simulink model "ABS_simp"  (R2015a)
settings: Solver=FixedStepDiscrete  StartTime=0.0  StopTime=1.0  FixedStep=1.0  RelTol=1e-3
libraries: simulink x2
settings Model: Creator=Teme  LastModifiedBy=Teme
settings DataIOCC: ExternalInput=Inputs_Safety_1_01062016175621  LoadExternalInput=on  SaveFormat=Structure  SaveState=on
settings RTWCC: Toolchain=Clang v3.1 | gmake (64-bit Mac)
settings GRTTargetCC: ExtMode=on

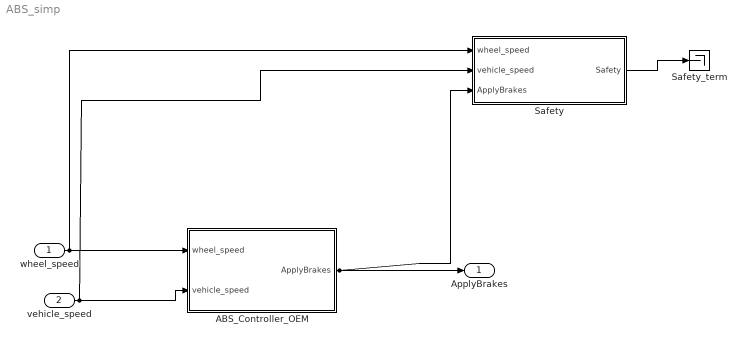
== system ABS_simp ==
  wheel_speed : Inport  SampleTime=0
  vehicle_speed : Inport  Port=2  SampleTime=0
  ABS_Controller_OEM : Subsystem
  Safety : Subsystem  TreatAsAtomicUnit=on  mask(Observer){AnnotationType=ensures, ObserverType=[]}
      mask prompts: AnnotationType "Type of annotation (pre/post...)"; ObserverType "Observer type"
      mask help:
      | Set an observer for the system.
      | The annotation type parameter sets the type of observer:
      | - requires : pre-condition
      | - ensures : post-condition
      | - assert : an assertion
      | - observer : the observer computes a special type of properties
      mask TypeOptions AnnotationType: ensures | requires | assert | observer
      mask Callback AnnotationType:
      | paramStr = get_param(gcb, 'MaskValues');
      | if strcmp(paramStr{1}(1),'o')
      | set_param(gcb,'MaskVisibilities',{'on';'on'});
      | paramStr{2} = 'ellipsoid';
      | set_param(gcb,'MaskValues',paramStr);
      | else
      | set_param(gcb,'MaskVisibilities',{'on';'off'});
      | end
      | clear paramStr;
      mask Callback ObserverType:
      | paramStr = get_param(gcb, 'MaskValues');
      | if strcmp(paramStr{1}(1),'o')
      | set_param(gcb,'MaskVisibilities',{'on';'on'});
      | paramStr{2} = 'ellipsoid';
      | set_param(gcb,'MaskValues',paramStr);
      | else
      | set_param(gcb,'MaskVisibilities',{'on';'off'});
      | end
      | clear paramStr;
      mask Display:
      | color('red')
      | text(0.5, 0.5, ['CoCoSpec: ''' get_param(gcb,'name') ''''], 'horizontalAlignment', 'center');
      | text(0.99, 0.03, '{\bf\fontsize{12}TO BE VERIFIED}', 'hor', 'right', 'ver', 'bottom', 'texmode', 'on');
  Safety_term : Terminator
  ApplyBrakes : Outport
  wires:
  wheel_speed/1 -> ABS_Controller_OEM/1(wheel_speed), Safety/1(wheel_speed)
  vehicle_speed/1 -> ABS_Controller_OEM/2(vehicle_speed), Safety/2(vehicle_speed)
  ABS_Controller_OEM/1(ApplyBrakes) -> ApplyBrakes/1, Safety/3(ApplyBrakes)
  Safety/1(Safety) -> Safety_term/1

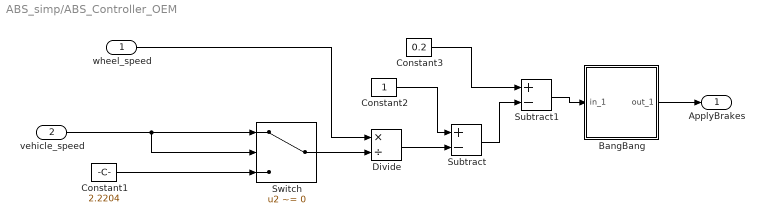
== system ABS_simp/ABS_Controller_OEM ==
  wheel_speed : Inport  SampleTime=0
  vehicle_speed : Inport  Port=2  SampleTime=0
  BangBang : Subsystem
  Constant1 : Constant  RequirementInfo={} %GIDa_68c76990_35e6_402e_a499_fea0c7d912d5  Value=2.2204  VectorParams1D=off
  Constant2 : Constant  RequirementInfo={} %GIDa_4a8a2e2c_8a4d_462f_a92b_c4449d5218d4  VectorParams1D=off
  Constant3 : Constant  RequirementInfo={} %GIDa_3f3dfe3e_fba3_4463_89e1_4e0ea70d5db5  Value=0.2  VectorParams1D=off
  Divide : Product  Inputs=*/
  Subtract : Sum  Inputs=+-
  Subtract1 : Sum  Inputs=+-
  Switch : Switch  RequirementInfo={} %GIDa_2bb70abf_1eef_45bd_b310_739057b34ef7  Criteria=u2 ~= 0
  ApplyBrakes : Outport
  wires:
  wheel_speed/1 -> Divide/1
  Constant1/1 -> Switch/3
  Divide/1 -> Subtract/2
  Constant2/1 -> Subtract/1
  Switch/1 -> Divide/2
  vehicle_speed/1 -> Switch/2, Switch/1
  Constant3/1 -> Subtract1/1
  Subtract1/1 -> BangBang/1(in_1)
  BangBang/1(out_1) -> ApplyBrakes/1
  Subtract/1 -> Subtract1/2

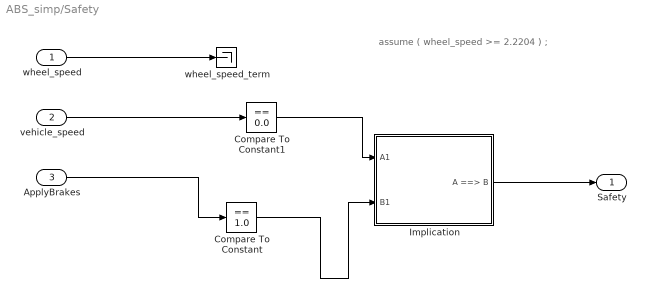
== system ABS_simp/Safety ==
  note: assume ( wheel_speed >= 2.2204 ) ;
  wheel_speed : Inport
  vehicle_speed : Inport  Port=2
  ApplyBrakes : Inport  Port=3
  Compare To Constant : simulink/Logic and Bit Operations/Compare To Constant  relop===  const=1.0  OutDataTypeStr=boolean
  Compare To Constant1 : simulink/Logic and Bit Operations/Compare To Constant  relop===  const=0.0  OutDataTypeStr=boolean
  Implication : Subsystem  mask(CoCoSim-Implies){}
      mask help: CoCoSim block for Logical Implication
      mask Display: disp(' ')
  wheel_speed_term : Terminator
  Safety : Outport
  wires:
  wheel_speed/1 -> wheel_speed_term/1
  vehicle_speed/1 -> Compare To Constant1/1
  ApplyBrakes/1 -> Compare To Constant/1
  Compare To Constant1/1 -> Implication/1(A1)
  Compare To Constant/1 -> Implication/2(B1)
  Implication/1(A ==> B) -> Safety/1

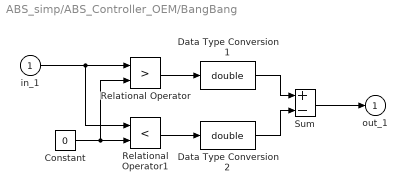
== system ABS_simp/ABS_Controller_OEM/BangBang ==
  in_1 : Inport
  Constant : Constant  Value=0
  Data Type Conversion1 : DataTypeConversion  OutDataTypeStr=double  SaturateOnIntegerOverflow=on  RndMeth=Zero
  Data Type Conversion2 : DataTypeConversion  OutDataTypeStr=double  SaturateOnIntegerOverflow=on  RndMeth=Zero
  Relational Operator : RelationalOperator  Operator=>  OutDataTypeStr=boolean  InputSameDT=on
  Relational Operator1 : RelationalOperator  Operator=<  OutDataTypeStr=boolean  InputSameDT=on
  Sum : Sum  Inputs=+-  SaturateOnIntegerOverflow=on  InputSameDT=on  OutDataTypeStr=Inherit: Same as first input
  out_1 : Outport  InitialOutput=0
  wires:
  in_1/1 -> Relational Operator1/1, Relational Operator/1
  Data Type Conversion2/1 -> Sum/2
  Constant/1 -> Relational Operator/2, Relational Operator1/2
  Relational Operator/1 -> Data Type Conversion1/1
  Data Type Conversion1/1 -> Sum/1
  Sum/1 -> out_1/1
  Relational Operator1/1 -> Data Type Conversion2/1

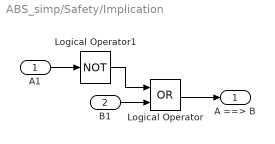
== system ABS_simp/Safety/Implication ==
  A1 : Inport
  B1 : Inport  Port=2
  Logical Operator : Logic  Operator=OR  AllPortsSameDT=off  OutDataTypeStr=boolean
  Logical Operator1 : Logic  Operator=NOT  AllPortsSameDT=off  OutDataTypeStr=boolean
  A ==> B : Outport
  wires:
  A1/1 -> Logical Operator1/1
  Logical Operator1/1 -> Logical Operator/1
  B1/1 -> Logical Operator/2
  Logical Operator/1 -> A ==> B/1
